simulink model "ex3b_model"  (R2013a)
settings: Solver=ode45  StartTime=0.0  StopTime=10.0  RelTol=1e-3
values from neighbouring files (symbols this model uses):
  q_0 = 0    [ex6.m]
  q_dot_0 = 0    [ex6.m]
settings Model: Creator=Brent  LastModifiedBy=Willdog

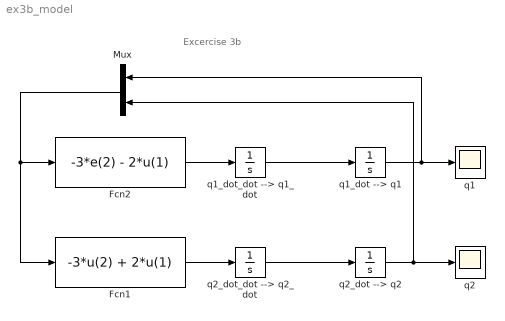
== system ex3b_model ==
  note: Excercise 3b
  Fcn1 : Fcn  Expr=-3*u(2) + 2*u(1)
  Fcn2 : Fcn  Expr=-3*e(2) - 2*u(1)
  Mux : Mux  Inputs=2
  q1 : Scope
  q1_dot --> q1 : Integrator  InitialCondition=q_0
  q1_dot_dot --> q1_dot : Integrator  InitialCondition=q_dot_0
  q2 : Scope
  q2_dot --> q2 : Integrator  InitialCondition=q_0
  q2_dot_dot --> q2_dot : Integrator  InitialCondition=q_dot_0
  wires:
  q1_dot_dot --> q1_dot/1 -> q1_dot --> q1/1
  q1_dot --> q1/1 -> Mux/1, q1/1
  q2_dot_dot --> q2_dot/1 -> q2_dot --> q2/1
  q2_dot --> q2/1 -> Mux/2, q2/1
  Fcn1/1 -> q2_dot_dot --> q2_dot/1
  Fcn2/1 -> q1_dot_dot --> q1_dot/1
  Mux/1 -> Fcn2/1, Fcn1/1
